simulink model "BikeModel"  (R2021b)
settings: Solver=FixedStepAuto  StartTime=0.0  StopTime=20  FixedStep=1e-4  RelTol=1e-3
values from neighbouring files (symbols this model uses):
  A = 1.446    [PlanarMotionBikeModel.m]
  B = BCD/(C*D)    [PatcejkaModel.m]    (also in PlanarMotionBikeModel.m = 1.408)
  BETA = 40    [PlanarMotionBikeModel.m]
  CDAMPING = 4000    [PlanarMotionBikeModel.m]
  CWHEEL = 0.15    [PlanarMotionBikeModel.m]
  D = Fz * (b1*Fz+b2)    (= 4400)    [PatcejkaModel.m]    (also in PlanarMotionBikeModel.m = 0.4)
  F = 0.3    [PlanarMotionBikeModel.m]
  g = 9.81    [PlanarMotionBikeModel.m]
  GAMMA = 75    [PlanarMotionBikeModel.m]
  H = b9*Fz + b10    (= 0)    [PatcejkaModel.m]    (also in PlanarMotionBikeModel.m = 0.4)
  HG = 0.53    [PlanarMotionBikeModel.m]
  HGC = 0.1    [PlanarMotionBikeModel.m]
  JWHEEL = 2.025    [PlanarMotionBikeModel.m]
  JXX_PRIME = 62.834    [PlanarMotionBikeModel.m]
  JZZPRIME = 1550    [PlanarMotionBikeModel.m]
  KR = 4e8    (= 400000000)    [PatcejkaModel.m]    (also in PlanarMotionBikeModel.m)
  KSPRING = 5000    [PlanarMotionBikeModel.m]
  KTL = 90000    [PatcejkaModel.m]    (also in PlanarMotionBikeModel.m)
  KTV = 110000    [PatcejkaModel.m]    (also in PlanarMotionBikeModel.m)
  M = 2200    [PlanarMotionBikeModel.m]
  ometa0 = v0/RWHEEL    (= 16.6666666667)    [PlanarMotionBikeModel.m]
  RWHEEL = 0.3    [PatcejkaModel.m]    (also in PlanarMotionBikeModel.m)
  T = 2.1/2    (= 1.05)    [PlanarMotionBikeModel.m]
  v0 = 5    [PlanarMotionBikeModel.m]
settings Model: Creator=Utente  LastModifiedBy=Utente

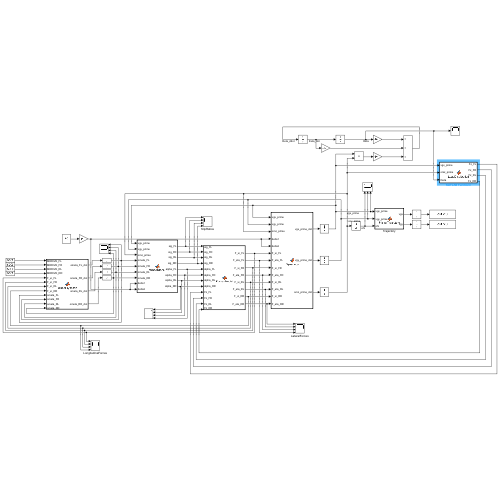
[thumbnail: Simulink's stored preview of the top-level diagram]
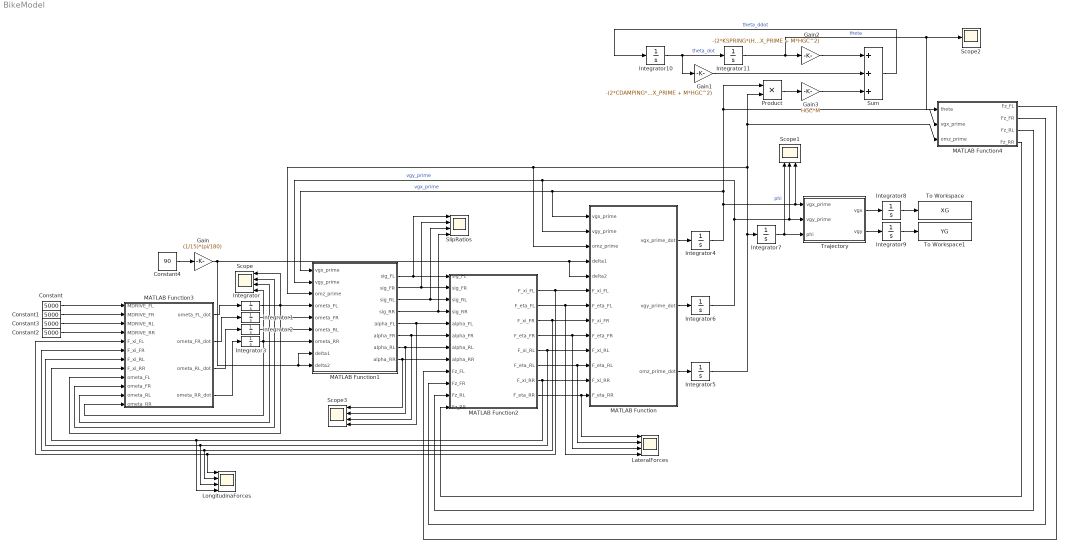
== system BikeModel ==
  Constant : Constant  Value=5000  SampleTime=0
  Constant1 : Constant  Value=5000
  Constant2 : Constant  Value=5000
  Constant3 : Constant  Value=5000
  Constant4 : Constant  Value=90
  Gain : Gain  Gain=(1/15)*(pi/180)
  Gain1 : Gain  Gain=-(2*CDAMPING*(H*cos(BETA) - (D/E)*F*cos(GAMMA))^2)/(JXX_PRIME + M*HGC^2)
  Gain2 : Gain  Gain=-(2*KSPRING*(H*cos(BETA) - (D/E)*F*cos(GAMMA))^2)/(JXX_PRIME + M*HGC^2)
  Gain3 : Gain  Gain=HGC*M
  Integrator{,1..3} (4 alike) : Integrator  InitialCondition=ometa0
  Integrator{5..11} (7 alike) : Integrator
  Integrator4 : Integrator  InitialCondition=v0
  LateralForces : Scope  NumInputPorts=4
  LongitudinaForces : Scope  NumInputPorts=4
  MATLAB Function : MATLAB Function  TreatAsAtomicUnit=on
  MATLAB Function1 : MATLAB Function  TreatAsAtomicUnit=on
  MATLAB Function2 : MATLAB Function  TreatAsAtomicUnit=on
  MATLAB Function3 : MATLAB Function  TreatAsAtomicUnit=on
  MATLAB Function4 : MATLAB Function  TreatAsAtomicUnit=on
  Product : Product
  Scope : Scope  NumInputPorts=4
  Scope1 : Scope  NumInputPorts=3
  Scope2 : Scope
  Scope3 : Scope  NumInputPorts=4
  SlipRatios : Scope  NumInputPorts=4
  Sum : Sum  Inputs=+++
  To Workspace : ToWorkspace  VariableName=XG  SampleTime=-1
      settings: Save2DSignal=2-D array (concatenate along first dimension)
  To Workspace1 : ToWorkspace  VariableName=YG  SampleTime=-1
      settings: Save2DSignal=2-D array (concatenate along first dimension)
  Trajectory : MATLAB Function  TreatAsAtomicUnit=on
  wires:
  MATLAB Function1/4(sig_RR) -> SlipRatios/4, MATLAB Function2/4(sig_RR)
  MATLAB Function1/1(sig_FL) -> SlipRatios/1, MATLAB Function2/1(sig_FL)
  MATLAB Function1/3(sig_RL) -> SlipRatios/3, MATLAB Function2/3(sig_RL)
  MATLAB Function1/5(alpha_FL) -> Scope3/4, MATLAB Function2/5(alpha_FL)
  MATLAB Function1/6(alpha_FR) -> Scope3/3, MATLAB Function2/6(alpha_FR)
  MATLAB Function1/7(alpha_RL) -> Scope3/2, MATLAB Function2/7(alpha_RL)
  MATLAB Function1/8(alpha_RR) -> Scope3/1, MATLAB Function2/8(alpha_RR)
  MATLAB Function2/1(F_xi_FL) -> MATLAB Function/6(F_xi_FL), LongitudinaForces/1, MATLAB Function3/5(F_xi_FL)
  MATLAB Function2/2(F_eta_FL) -> LateralForces/4, MATLAB Function/7(F_eta_FL)
  MATLAB Function2/3(F_xi_FR) -> MATLAB Function/8(F_xi_FR), MATLAB Function3/6(F_xi_FR), LongitudinaForces/2
  MATLAB Function2/4(F_eta_FR) -> LateralForces/3, MATLAB Function/9(F_eta_FR)
  MATLAB Function2/5(F_xi_RL) -> MATLAB Function/10(F_xi_RL), MATLAB Function3/7(F_xi_RL), LongitudinaForces/3
  MATLAB Function2/6(F_eta_RL) -> LateralForces/2, MATLAB Function/11(F_eta_RL)
  MATLAB Function2/7(F_xi_RR) -> MATLAB Function/12(F_xi_RR), MATLAB Function3/8(F_xi_RR), LongitudinaForces/4
  MATLAB Function2/8(F_eta_RR) -> LateralForces/1, MATLAB Function/13(F_eta_RR)
  MATLAB Function3/1(ometa_FL_dot) -> Integrator/1
  MATLAB Function3/2(ometa_FR_dot) -> Integrator1/1
  MATLAB Function3/3(ometa_RL_dot) -> Integrator2/1
  MATLAB Function3/4(ometa_RR_dot) -> Integrator3/1
  Integrator/1 -> Scope/1, MATLAB Function3/9(ometa_FL), MATLAB Function1/4(ometa_FL)
  Integrator1/1 -> MATLAB Function3/10(ometa_FR), MATLAB Function1/5(ometa_FR), Scope/2
  Integrator2/1 -> MATLAB Function3/11(ometa_RL), MATLAB Function1/6(ometa_RL), Scope/3
  Integrator3/1 -> MATLAB Function3/12(ometa_RR), MATLAB Function1/7(ometa_RR), Scope/4
  MATLAB Function/3(omz_prime_dot) -> Integrator5/1
  MATLAB Function/2(vgy_prime_dot) -> Integrator6/1
  MATLAB Function/1(vgx_prime_dot) -> Integrator4/1
  Integrator5/1 -> Integrator7/1, MATLAB Function/3(omz_prime), MATLAB Function1/3(omz_prime), Product/2, MATLAB Function4/3(omz_prime)
  Integrator6/1 -> Trajectory/2(vgy_prime), Scope1/2, MATLAB Function/2(vgy_prime), MATLAB Function1/2(vgy_prime)  "vgy_prime"
  Integrator4/1 -> MATLAB Function/1(vgx_prime), MATLAB Function1/1(vgx_prime), Product/1, MATLAB Function4/2(vgx_prime), Trajectory/1(vgx_prime), Scope1/3  "vgx_prime"
  Constant/1 -> MATLAB Function3/1(MDRIVE_FL)
  Constant1/1 -> MATLAB Function3/2(MDRIVE_FR)
  Constant3/1 -> MATLAB Function3/3(MDRIVE_RL)
  Constant2/1 -> MATLAB Function3/4(MDRIVE_RR)
  Constant4/1 -> Gain/1
  Integrator8/1 -> To Workspace/1
  Integrator9/1 -> To Workspace1/1
  Trajectory/1(vgx) -> Integrator8/1
  Integrator7/1 -> Scope1/1, Trajectory/3(phi)  "phi"
  Trajectory/2(vgy) -> Integrator9/1
  MATLAB Function1/2(sig_FR) -> SlipRatios/2, MATLAB Function2/2(sig_FR)
  Gain/1 -> MATLAB Function1/8(delta1), MATLAB Function1/9(delta2), MATLAB Function/4(delta1), MATLAB Function/5(delta2)
  Sum/1 -> Integrator10/1  "theta_ddot"
  Integrator10/1 -> Integrator11/1, Gain1/1  "theta_dot"
  Integrator11/1 -> MATLAB Function4/1(theta), Scope2/1, Gain2/1  "theta"
  Gain2/1 -> Sum/1
  Product/1 -> Gain3/1
  Gain3/1 -> Sum/3
  Gain1/1 -> Sum/2
  MATLAB Function4/1(Fz_FL) -> MATLAB Function2/9(Fz_FL)
  MATLAB Function4/2(Fz_FR) -> MATLAB Function2/10(Fz_FR)
  MATLAB Function4/3(Fz_RL) -> MATLAB Function2/11(Fz_RL)
  MATLAB Function4/4(Fz_RR) -> MATLAB Function2/12(Fz_RR)

== matlab function BikeModel/MATLAB Function2 ==
  data: F_xi_FL output; F_eta_FL output; F_xi_FR output; F_eta_FR output; sig_FL input; sig_FR input; sig_RL input; sig_RR input; alpha_FL input; alpha_FR input; alpha_RL input; alpha_RR input; Fz_FL input; Fz_FR input; Fz_RL input; Fz_RR input; F_xi_RL output; F_eta_RL output; F_xi_RR output; F_eta_RR output; CWHEEL parameter; RWHEEL parameter; KTL parameter; KR parameter; KTV parameter
function [F_xi_FL, F_eta_FL, F_xi_FR, F_eta_FR, F_xi_RL, F_eta_RL, F_xi_RR, F_eta_RR] = ForcesModel(sig_FL, sig_FR, sig_RL, sig_RR, ...
          alpha_FL, alpha_FR, alpha_RL, alpha_RR, Fz_FL, Fz_FR, Fz_RL, Fz_RR, CWHEEL, RWHEEL, KTL, KR, KTV)

F_xi_FL = (6*RWHEEL*KTL*Fz_FL)*sig_FL/(CWHEEL*KR);
F_xi_FR = (6*RWHEEL*KTL*Fz_FR)*sig_FR/(CWHEEL*KR);
F_xi_RL = (6*RWHEEL*KTL*Fz_RL)*sig_RL/(CWHEEL*KR);
F_xi_RR = (6*RWHEEL*KTL*Fz_RR)*sig_RR/(CWHEEL*KR);

F_eta_FL = (6*RWHEEL*KTV*Fz_FL*alpha_FL)/(CWHEEL*KR);
F_eta_FR = (6*RWHEEL*KTV*Fz_FR*alpha_FR)/(CWHEEL*KR);
F_eta_RL = (6*RWHEEL*KTV*Fz_RL*alpha_RL)/(CWHEEL*KR);
F_eta_RR = (6*RWHEEL*KTV*Fz_RR*alpha_RR)/(CWHEEL*KR);

end

== matlab function BikeModel/MATLAB Function3 ==
  data: MDRIVE_FL input; ometa_FL_dot output; MDRIVE_FR input; MDRIVE_RL input; MDRIVE_RR input; F_xi_FL input; F_xi_FR input; F_xi_RL input; F_xi_RR input; ometa_FR_dot output; JWHEEL parameter; ometa_RL_dot output; ometa_RR_dot output; RWHEEL parameter; ometa_FL input; ometa_FR input; ometa_RL input; ometa_RR input
function [ometa_FL_dot, ometa_FR_dot, ometa_RL_dot, ometa_RR_dot] = WheelDynamic(MDRIVE_FL, MDRIVE_FR, MDRIVE_RL, MDRIVE_RR, F_xi_FL, F_xi_FR, F_xi_RL, F_xi_RR, JWHEEL, RWHEEL, ometa_FL, ometa_FR, ometa_RL, ometa_RR)


ometa_FL_dot = (1/JWHEEL)*(MDRIVE_FL/ometa_FL - RWHEEL*F_xi_FL);
ometa_FR_dot = (1/JWHEEL)*(MDRIVE_FR/ometa_FR - RWHEEL*F_xi_FR);
ometa_RL_dot = (1/JWHEEL)*(MDRIVE_RL/ometa_RL - RWHEEL*F_xi_RL);
ometa_RR_dot = (1/JWHEEL)*(MDRIVE_RR/ometa_RR - RWHEEL*F_xi_RR);

end

== matlab function BikeModel/Trajectory ==
  data: vgx_prime input; vgx output; vgy_prime input; phi input; vgy output
function [vgx,vgy] = PlanarTrajectory(vgx_prime, vgy_prime, phi)

MROT = [[cos(phi) -sin(phi)];
        [sin(phi) cos(phi)]];

state_prime = [vgx_prime, vgy_prime]';

state = MROT*state_prime;

vgx = state(1);
vgy = state(2);
end

== matlab function BikeModel/MATLAB Function4 ==
  data: theta input; Fz_FL output; vgx_prime input; omz_prime input; Fz_FR output; g parameter; HGC parameter; HG parameter; T parameter; M parameter; Fz_RL output; Fz_RR output
function [Fz_FL, Fz_FR, Fz_RL, Fz_RR] = LoadDistribution(theta, vgx_prime, omz_prime, g, HGC, HG, T, M)

Fcent = M*omz_prime*vgx_prime;

Fz_FL = (M*g*(1 + 2*HGC*theta/(2*T)) + Fcent*(HG/2*T))/2;
Fz_RL = (M*g*(1 + 2*HGC*theta/(2*T)) + Fcent*(HG/2*T))/2;
Fz_FR = (M*g*(1 - 2*HGC*theta/(2*T)) - Fcent*(HG/2*T))/2;
Fz_RR = (M*g*(1 - 2*HGC*theta/(2*T)) - Fcent*(HG/2*T))/2;

end

== matlab function BikeModel/MATLAB Function1 ==
  data: vgx_prime input; vgy_prime input; omz_prime input; sig_FL output; sig_FR output; sig_RL output; sig_RR output; RWHEEL parameter; ometa_FL input; ometa_FR input; ometa_RL input; ometa_RR input; delta1 input; delta2 input; A parameter; B parameter; alpha_FL output; alpha_FR output; alpha_RL output; alpha_RR output; T parameter
function [sig_FL, sig_FR, sig_RL, sig_RR, alpha_FL, alpha_FR, alpha_RL, alpha_RR] = WheelModel(vgx_prime, vgy_prime, omz_prime, RWHEEL, ometa_FL, ...
          ometa_FR, ometa_RL, ometa_RR, delta1, delta2, A, B, T)

vFL = (vgx_prime - T*omz_prime)*cos(delta1) + (vgy_prime + A*omz_prime)*sin(delta1);
vFR = (vgx_prime + T*omz_prime)*cos(delta2) + (vgy_prime + A*omz_prime)*sin(delta2);
vRL = (vgx_prime - T*omz_prime);
vRR = (vgx_prime + T*omz_prime);

sig_FL = (1 - vFL/(RWHEEL*ometa_FL))*100;
sig_FR = (1 - vFR/(RWHEEL*ometa_FR))*100;
sig_RL = (1 - vRL/(RWHEEL*ometa_RL))*100;
sig_RR = (1 - vRR/(RWHEEL*ometa_RR))*100;

alpha_FL = (delta1 - atan(( vgy_prime + A*omz_prime)/(vgx_prime - T*omz_prime)))*(180/pi);
alpha_FR = (delta2 - atan(( vgy_prime + A*omz_prime)/(vgx_prime + T*omz_prime)))*(180/pi);
alpha_RL =          (atan((-vgy_prime + B*omz_prime)/(vgx_prime - T*omz_prime)))*(180/pi);
alpha_RR =          (atan((-vgy_prime + B*omz_prime)/(vgx_prime + T*omz_prime)))*(180/pi);


end

== matlab function BikeModel/MATLAB Function ==
  data: vgx_prime input; vgy_prime input; omz_prime input; delta1 input; delta2 input; JZZPRIME parameter; M parameter; A parameter; vgx_prime_dot output; vgy_prime_dot output; omz_prime_dot output; B parameter; T parameter; F_xi_FL input; F_eta_FL input; F_xi_FR input; F_eta_FR input; F_xi_RL input; F_eta_RL input; F_xi_RR input; F_eta_RR input
function [vgx_prime_dot, vgy_prime_dot, omz_prime_dot] = Dynamics(vgx_prime, vgy_prime, omz_prime, delta1, delta2, JZZPRIME, M, A, B, T,...
          F_xi_FL, F_eta_FL, F_xi_FR, F_eta_FR, F_xi_RL, F_eta_RL, F_xi_RR, F_eta_RR) 

F_x_FL = F_xi_FL*cos(delta1) - F_eta_FL*sin(delta1);
F_y_FL = F_xi_FL*sin(delta1) + F_eta_FL*cos(delta1);
F_x_FR = F_xi_FR*cos(delta2) - F_eta_FR*sin(delta2);
F_y_FR = F_xi_FR*sin(delta2) + F_eta_FR*cos(delta2);
F_x_RL = F_xi_RL;
F_y_RL = F_eta_RL;
F_x_RR = F_xi_RR;
F_y_RR = F_eta_RR;

vgx_prime_dot =  vgy_prime*omz_prime + (1/M)*(F_x_FL + F_x_FR + F_x_RL + F_x_RR);
vgy_prime_dot = -vgx_prime*omz_prime + (1/M)*(F_y_FL + F_y_FR + F_y_RL + F_y_RR);
omz_prime_dot = (1/JZZPRIME)*( A*(F_y_FL + F_y_FR) - B*(F_y_RL + F_y_RR) ...
                 -T*F_x_FL + T*F_x_FR - T*F_x_RL + T*F_x_RR);

end
